simulink model "component_2D757F51390CB116_draft_harness"  (R2024b)
settings: Solver=FixedStepDiscrete  StartTime=0.0  StopTime=EV_stop  FixedStep=EV_dt  RelTol=1e-3
libraries: SignalEditorBlockLib x1
settings Model: Creator=menda  LastModifiedBy=menda

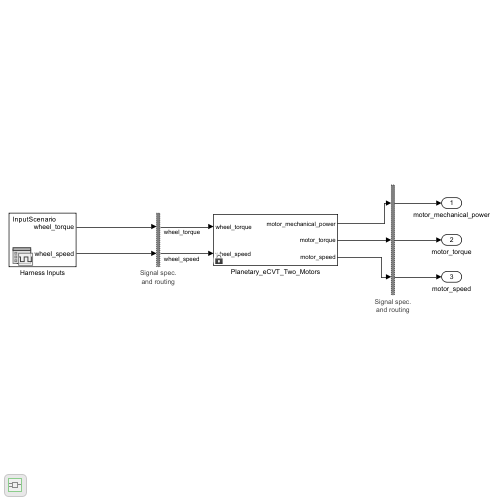
[thumbnail: Simulink's stored preview of the top-level diagram]
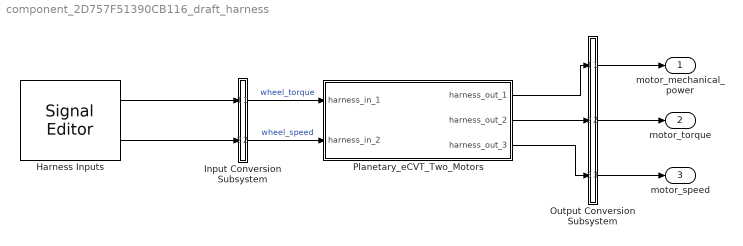
== system component_2D757F51390CB116_draft_harness ==
  Harness Inputs : SignalEditorBlockLib/Signal Editor  FileName=C:\Users\menda\OneDrive\Documentos\HackatonSAE\slprj\mbd_agent\test\EV_Backward_Baseline\component_2D757F51390CB116_draft_harness_HarnessInputs.mat  ActiveScenario=InputScenario  ActiveSignal=wheel_speed  IsBus=off  OutputBusObjectStr=Bus: BusObject  SampleTime=[0,1]  Interpolate=off  ZeroCross=off  OutputAfterFinalValue=Setting to zero  Unit=inherit  PreserveSignalName=on  ApplySigPropsToAllScenarios=on  ApplySigPropsToAllSignals=off
  Input Conversion Subsystem : Subsystem  Tag=__SLT_ICS__  Description=|
      | Signal spec.
      | and routing
      settings: AttributesFormatString=%<Description>
  Output Conversion Subsystem : Subsystem  Tag=__SLT_OCS__  Description=|
      | Signal spec.
      | and routing
      settings: AttributesFormatString=%<Description>
  Planetary_eCVT_Two_Motors : Subsystem  Tag=__SL_testing_harness_stub_
  motor_mechanical_power : Outport
  motor_torque : Outport  Port=2
  motor_speed : Outport  Port=3
  wires:
  Harness Inputs/1 -> Input Conversion Subsystem/1(Inport_1)
  Harness Inputs/2 -> Input Conversion Subsystem/2(Inport_2)
  Output Conversion Subsystem/1(Outport_1) -> motor_mechanical_power/1
  Output Conversion Subsystem/2(Outport_2) -> motor_torque/1
  Output Conversion Subsystem/3(Outport_3) -> motor_speed/1
  Input Conversion Subsystem/1(Outport_1) -> Planetary_eCVT_Two_Motors/1(harness_in_1)  "wheel_torque"
  Input Conversion Subsystem/2(Outport_2) -> Planetary_eCVT_Two_Motors/2(harness_in_2)  "wheel_speed"
  Planetary_eCVT_Two_Motors/1(harness_out_1) -> Output Conversion Subsystem/1(Inport_1)
  Planetary_eCVT_Two_Motors/2(harness_out_2) -> Output Conversion Subsystem/2(Inport_2)
  Planetary_eCVT_Two_Motors/3(harness_out_3) -> Output Conversion Subsystem/3(Inport_3)

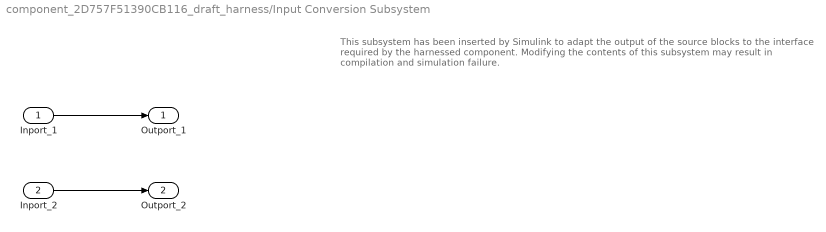
== system component_2D757F51390CB116_draft_harness/Input Conversion Subsystem ==
  note: This subsystem has been inserted by Simulink to adapt the output of the source blocks to the interface required by the harnessed component.
      |  Modifying the contents of this subsystem may result in compilation and simulation failure.
  Inport_1 : Inport
  Inport_2 : Inport  Port=2
  Outport_1 : Outport
  Outport_2 : Outport  Port=2
  wires:
  Inport_1/1 -> Outport_1/1
  Inport_2/1 -> Outport_2/1

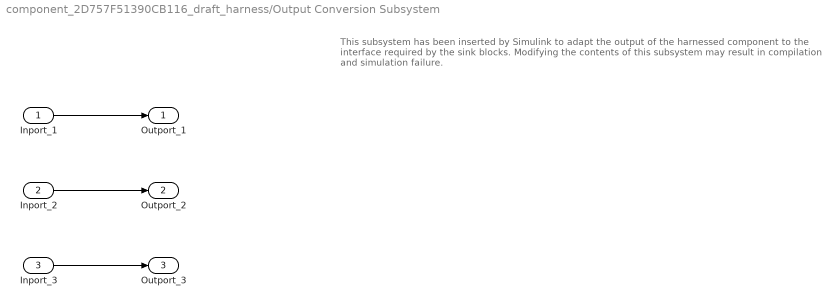
== system component_2D757F51390CB116_draft_harness/Output Conversion Subsystem ==
  note: This subsystem has been inserted by Simulink to adapt the output of the harnessed component to the interface required by the sink blocks.
      |  Modifying the contents of this subsystem may result in compilation and simulation failure.
  Inport_1 : Inport
  Inport_2 : Inport  Port=2
  Inport_3 : Inport  Port=3
  Outport_1 : Outport
  Outport_2 : Outport  Port=2
  Outport_3 : Outport  Port=3
  wires:
  Inport_1/1 -> Outport_1/1
  Inport_2/1 -> Outport_2/1
  Inport_3/1 -> Outport_3/1

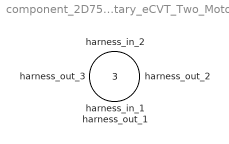
== system component_2D757F51390CB116_draft_harness/Planetary_eCVT_Two_Motors ==
  harness_in_1 : Inport
  harness_in_2 : Inport  Port=2
  harness_out_1 : Outport
  harness_out_2 : Outport  Port=2
  harness_out_3 : Outport  Port=3
